simulink model "Sanepa_overall_model0x2810x29"  (R2024b)
settings: Solver=VariableStepAuto  StartTime=0.0  StopTime=0.7  RelTol=1e-3
undefined symbols (not defined in the file or in its folder): D11, Delta, DiscIntNeverNeededParam
libraries: spsSeriesRLCLoadLib x69, spsThreePhaseTransformerTwoWindingsLib x23, spsThreePhasePISectionLineLib x18, spsRMSLib x6, spsThreePhaseSeriesRLCBranchLib x4, spsThreePhaseVIMeasurementLib x3, spsCurrentMeasurementLib x3, spsVoltageMeasurementLib x3, spsGroundLib x2, spsThreePhaseBreakerLib x2, spsabctodq0Lib x1, spsdq0toabcLib x1
(part 2 of 2)

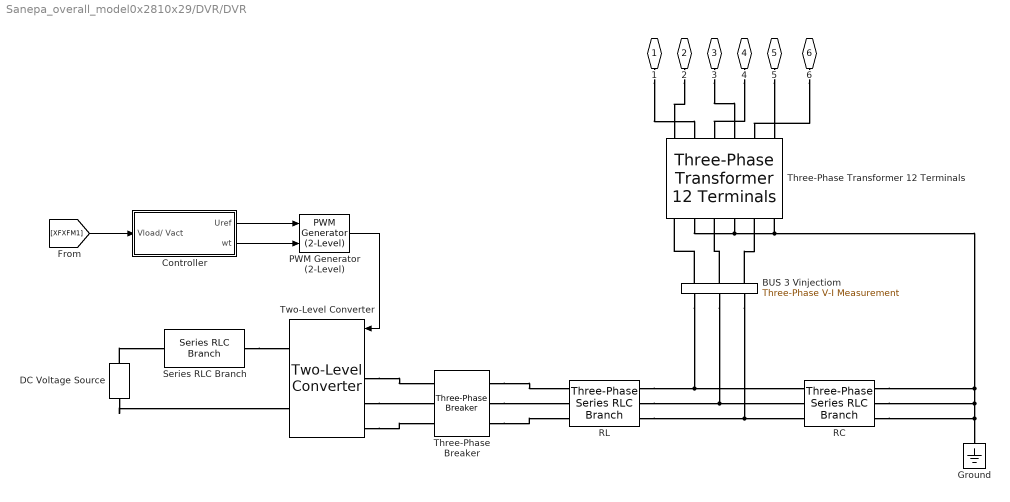
== system Sanepa_overall_model0x2810x29/DVR/DVR ==
  BUS 3 Vinjectiom : spsThreePhaseVIMeasurementLib/Three-Phase V-I Measurement  VoltageMeasurement=phase-to-ground  SetLabelV=on  LabelV=Vinj  Vpu=on  VpuLL=off  CurrentMeasurement=yes  SetLabelI=on  LabelI=Iinj  Ipu=on  Pbase=1e6  Vbase=11000  OutputType=Complex  PhasorSimulation=off  PSBequivalent=0
  Controller : Subsystem
  DC Voltage Source : spsDCVoltageSourceLib/DC Voltage Source  Amplitude=3000  Measurements=None
  Ground : spsGroundLib/Ground  LConnTagsString=a
  PWM Generator (2-Level) : spsPWMGenerator2LevelLib/PWM Generator (2-Level)  ModulatorType=Three-phase bridge (6 pulses)  ModulatorMode=Synchronized  Fc=27*60  Pc=90  nF=2250  MinMax="[ -1  1 ]"  SamplingTechnique=Natural  ModulatingSignals=off  m=0.8  Freq=60  Phase=0  Ts=50e-6  ShowCarrierOutport=off
  RC : spsThreePhaseSeriesRLCBranchLib/Three-Phase Series RLC Branch  LConnTagsString=A|B|C  RConnTagsString=A|B|C  BranchType=RC  Resistance=1  Inductance=1e-3  Capacitance=50e-7  Measurements=None
  RL : spsThreePhaseSeriesRLCBranchLib/Three-Phase Series RLC Branch  LConnTagsString=A|B|C  RConnTagsString=A|B|C  BranchType=L  Resistance=1  Inductance=1e-1  Capacitance=1e-6  Measurements=None
  Series RLC Branch : spsSeriesRLCBranchLib/Series RLC Branch  LConnTagsString=__new0  RConnTagsString=__new0  BranchType=R  Resistance=0.1  Inductance=1e-3  SetiL0=off  InitialCurrent=0  Capacitance=1e-6  Setx0=off  InitialVoltage=0  Measurements=None
  Three-Phase Breaker : spsThreePhaseBreakerLib/Three-Phase Breaker  InitialState=open  SwitchA=on  SwitchB=on  SwitchC=on  SwitchTimes=0  External=off  BreakerResistance=0.01  SnubberResistance=1e6  SnubberCapacitance=inf  Measurements=None
  Three-Phase Transformer 12 Terminals : spsThreePhaseTransformer12TerminalsLib/Three-Phase Transformer 12 Terminals  RatedPower=[ 100e3 50 ]  Winding1="[ 100 0.00001  0.0003 ]"  Winding2=[ 1000 0.00001 0.0003 ]  RmXm=[ 200 200 ]
  Two-Level Converter : spsTwoLevelConverterLib/Two-Level Converter  ModelType=Switching devices  Ron=1e-3  Rs=1e6  Cs=inf  Vforward=[0,0]  Ron_Diode=1e-3  Rs_Diode=1e6  Cs_Diode=inf  Vf_Diode=1e-3  Rs_CurrentSource=inf  Ron_ACsource=1e-3
  1 : PMIOPort  Tag=PMCPort  Side=Left
  2 : PMIOPort  Tag=PMCPort  Port=2  Side=Left
  3 : PMIOPort  Tag=PMCPort  Port=3  Side=Left
  4 : PMIOPort  Tag=PMCPort  Port=4  Side=Left
  5 : PMIOPort  Tag=PMCPort  Port=5  Side=Left
  6 : PMIOPort  Tag=PMCPort  Port=6  Side=Left
  wires:
  PWM Generator (2-Level)/1 -> Two-Level Converter/1
  Controller/1(Uref) -> PWM Generator (2-Level)/1
  Controller/2(wt) -> PWM Generator (2-Level)/2
  [XFXFM1] -> Controller/1(Vload/ Vact)
  connections:
  DC Voltage Source/RConn1 -- Series RLC Branch/LConn1
  DC Voltage Source/LConn1 -- Two-Level Converter/RConn2
  Series RLC Branch/RConn1 -- Two-Level Converter/RConn1
  Two-Level Converter/LConn1 -- Three-Phase Breaker/LConn1
  Two-Level Converter/LConn2 -- Three-Phase Breaker/LConn2
  Two-Level Converter/LConn3 -- Three-Phase Breaker/LConn3
  Three-Phase Breaker/RConn1 -- RL/LConn1
  Three-Phase Breaker/RConn2 -- RL/LConn2
  Three-Phase Breaker/RConn3 -- RL/LConn3
  RL/RConn1 -- BUS 3 Vinjectiom/LConn1 -- RC/LConn1
  RL/RConn2 -- BUS 3 Vinjectiom/LConn2 -- RC/LConn2
  RL/RConn3 -- BUS 3 Vinjectiom/LConn3 -- RC/LConn3
  Three-Phase Transformer 12 Terminals/LConn2 -- Three-Phase Transformer 12 Terminals/LConn4 -- RC/RConn3 -- Ground/LConn1 -- RC/RConn2 -- RC/RConn1 -- Three-Phase Transformer 12 Terminals/LConn6
  BUS 3 Vinjectiom/RConn1 -- Three-Phase Transformer 12 Terminals/LConn1
  BUS 3 Vinjectiom/RConn2 -- Three-Phase Transformer 12 Terminals/LConn3
  BUS 3 Vinjectiom/RConn3 -- Three-Phase Transformer 12 Terminals/LConn5
  1/RConn1 -- Three-Phase Transformer 12 Terminals/RConn2
  2/RConn1 -- Three-Phase Transformer 12 Terminals/RConn1
  3/RConn1 -- Three-Phase Transformer 12 Terminals/RConn4
  4/RConn1 -- Three-Phase Transformer 12 Terminals/RConn3
  5/RConn1 -- Three-Phase Transformer 12 Terminals/RConn6
  6/RConn1 -- Three-Phase Transformer 12 Terminals/RConn5

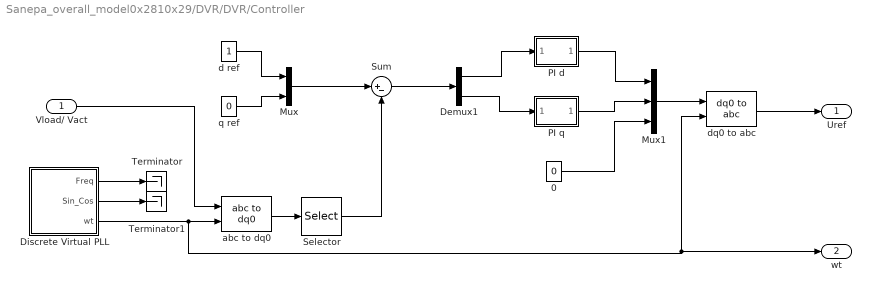
== system Sanepa_overall_model0x2810x29/DVR/DVR/Controller ==
  Vload/ Vact : Inport
  0 : Constant  Value=0
  Demux1 : Demux  Outputs=2
  Discrete Virtual PLL : Subsystem  DialogController=POWERSYS.PowerSysDialog  mask(Discrete Virtual PLL){Freq=50, Phase=30, Ts=50e-6}
      mask prompts: Freq "Frequency (Hz):"; Phase "Phase (degrees):"; Ts "Sample time:"
      mask help:
      | This virtual PLL has no input signal. The block simulates the outputs of an actual PLL by  using the parameters specified in the mask.
      |
      | Output 1: Frequency (Hz)
      | Output 2: Vectorized output  [sin(wt)  cos(wt)]
      | Output 3: wt in rad/s (varying from 0 to 2*pi)
      mask init:
      | power_initmask();
      mask Display: disp('')
  Mux : Mux  Inputs=2
  Mux1 : Mux  Inputs=3
  "PI d " : Subsystem  DialogController=POWERSYS.PowerSysDialog  mask(Discrete PI Controller){Kp=35, Ki=120, Par_Limits=[inf -inf], Init=0, Ts=50e-6}
      mask prompts: Kp "Proportional gain (Kp):"; Ki "Integral gain (Ki):"; Par_Limits "Output limits: [ Upper   Lower ]"; Init "Output initial value:"; Ts "Sample time:"
      mask help: This block implements a discrete PI controller.
      mask init:
      | UpperLimit=Par_Limits(1);
      | LowerLimit=Par_Limits(2);
      | power_initmask();
      mask Display: disp('PI');
  PI q : Subsystem  DialogController=POWERSYS.PowerSysDialog  mask(Discrete PI Controller){Kp=20, Ki=220, Par_Limits=[inf -inf], Init=0, Ts=50e-6}
      mask prompts: Kp "Proportional gain (Kp):"; Ki "Integral gain (Ki):"; Par_Limits "Output limits: [ Upper   Lower ]"; Init "Output initial value:"; Ts "Sample time:"
      mask help: This block implements a discrete PI controller.
      mask init:
      | UpperLimit=Par_Limits(1);
      | LowerLimit=Par_Limits(2);
      | power_initmask();
      mask Display: disp('PI');
  Selector : Selector  InputPortWidth=3  IndexOptions=Index vector (dialog)  Indices=[1 2]  OutputSizes=1
  Sum : Sum  Inputs=|+-
  Terminator : Terminator
  Terminator1 : Terminator
  abc to dq0 : spsabctodq0Lib/abc to dq0  Alignment=90 degrees behind phase A axis
  d ref : Constant
  dq0 to abc : spsdq0toabcLib/dq0 to abc  Alignment=90 degrees behind phase A axis
  q ref : Constant  Value=0
  Uref : Outport  VectorParamsAs1DForOutWhenUnconnected=off
  wt : Outport  Port=2  VectorParamsAs1DForOutWhenUnconnected=off
  wires:
  Discrete Virtual PLL/1(Freq) -> Terminator/1
  Discrete Virtual PLL/2(Sin_Cos) -> Terminator1/1
  Discrete Virtual PLL/3(wt) -> wt/1, dq0 to abc/2, abc to dq0/2
  Vload/ Vact/1 -> abc to dq0/1
  abc to dq0/1 -> Selector/1
  Selector/1 -> Sum/2
  Mux/1 -> Sum/1
  q ref/1 -> Mux/2
  d ref/1 -> Mux/1
  Sum/1 -> Demux1/1
  Demux1/1 -> "PI d "/1(Error)
  Demux1/2 -> PI q/1(Error)
  "PI d "/1(Out) -> Mux1/1
  PI q/1(Out) -> Mux1/2
  Mux1/1 -> dq0 to abc/1
  dq0 to abc/1 -> Uref/1
  0/1 -> Mux1/3

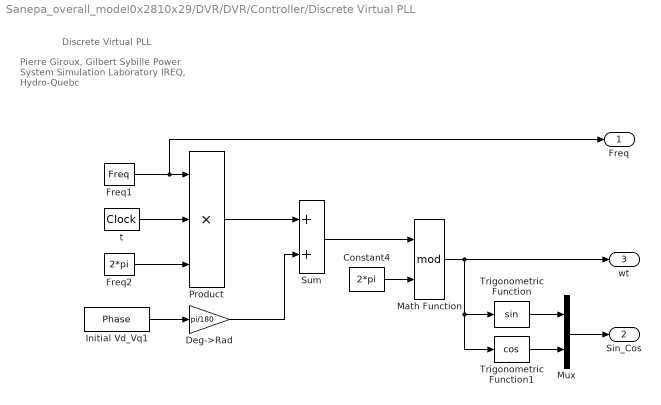
== system Sanepa_overall_model0x2810x29/DVR/DVR/Controller/Discrete Virtual PLL ==
  note: Pierre Giroux, Gilbert Sybille
      | Power System Simulation Laboratory
      | IREQ, Hydro-Quebc
  note: Discrete Virtual PLL
  Constant4 : Constant  Value=2*pi
  Deg->Rad : Gain  Gain=pi/180  SaturateOnIntegerOverflow=on  OutDataTypeStr=Inherit: Same as input  ParamDataTypeStr=Inherit: Same as input
  Freq1 : Constant  Value=Freq
  Freq2 : Constant  Value=2*pi
  Initial Vd_Vq1 : Constant  Value=Phase
  Math Function : Math  Operator=mod  SignedPower=on
  Mux : Mux  Inputs=2
  Product : Product  Inputs=***  InputSameDT=on  SaturateOnIntegerOverflow=on  OutDataTypeStr=Inherit: Same as first input
  Sum : Sum  InputSameDT=on  SaturateOnIntegerOverflow=on  OutDataTypeStr=Inherit: Same as first input
  Trigonometric Function : Trigonometry
  Trigonometric Function1 : Trigonometry  Operator=cos
  t : DigitalClock  SampleTime=Ts
  Freq : Outport  VectorParamsAs1DForOutWhenUnconnected=off
  Sin_Cos : Outport  Port=2  VectorParamsAs1DForOutWhenUnconnected=off
  wt : Outport  Port=3  VectorParamsAs1DForOutWhenUnconnected=off
  wires:
  Sum/1 -> Math Function/1
  t/1 -> Product/2
  Freq2/1 -> Product/3
  Freq1/1 -> Product/1, Freq/1
  Deg->Rad/1 -> Sum/2
  Initial Vd_Vq1/1 -> Deg->Rad/1
  Product/1 -> Sum/1
  Constant4/1 -> Math Function/2
  Math Function/1 -> wt/1, Trigonometric Function1/1, Trigonometric Function/1
  Trigonometric Function/1 -> Mux/1
  Trigonometric Function1/1 -> Mux/2
  Mux/1 -> Sin_Cos/1

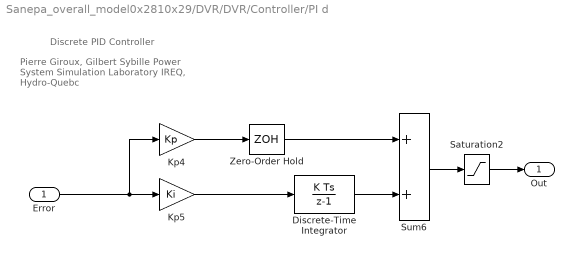
== system Sanepa_overall_model0x2810x29/DVR/DVR/Controller/PI d  ==
  note: Discrete PID Controller
  note: Pierre Giroux, Gilbert Sybille
      | Power System Simulation Laboratory
      | IREQ, Hydro-Quebc
  Error : Inport  SampleTime=Ts
  Discrete-Time Integrator : DiscreteIntegrator  InitialCondition=Init  SampleTime=Ts  LimitOutput=on  UpperSaturationLimit=UpperLimit  LowerSaturationLimit=LowerLimit  ICPrevOutput=DiscIntNeverNeededParam  ICPrevScaledInput=DiscIntNeverNeededParam
  Kp4 : Gain  Gain=Kp  SaturateOnIntegerOverflow=on  SampleTime=Ts  OutDataTypeStr=Inherit: Same as input  ParamDataTypeStr=Inherit: Same as input
  Kp5 : Gain  Gain=Ki  SaturateOnIntegerOverflow=on  SampleTime=Ts  OutDataTypeStr=Inherit: Same as input  ParamDataTypeStr=Inherit: Same as input
  Saturation2 : Saturate  UpperLimit=UpperLimit  LowerLimit=LowerLimit  SampleTime=Ts
  Sum6 : Sum  InputSameDT=on  SaturateOnIntegerOverflow=on  SampleTime=Ts  OutDataTypeStr=Inherit: Same as first input
  Zero-Order Hold : ZeroOrderHold  SampleTime=Ts
  Out : Outport  SampleTime=Ts  InitialOutput=0  VectorParamsAs1DForOutWhenUnconnected=off
  wires:
  Zero-Order Hold/1 -> Sum6/1
  Saturation2/1 -> Out/1
  Discrete-Time Integrator/1 -> Sum6/2
  Kp4/1 -> Zero-Order Hold/1
  Kp5/1 -> Discrete-Time Integrator/1
  Sum6/1 -> Saturation2/1
  Error/1 -> Kp5/1, Kp4/1

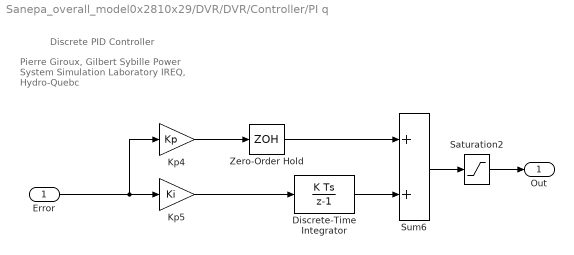
== system Sanepa_overall_model0x2810x29/DVR/DVR/Controller/PI q ==
  note: Pierre Giroux, Gilbert Sybille
      | Power System Simulation Laboratory
      | IREQ, Hydro-Quebc
  note: Discrete PID Controller
  Error : Inport  SampleTime=Ts
  Discrete-Time Integrator : DiscreteIntegrator  InitialCondition=Init  SampleTime=Ts  LimitOutput=on  UpperSaturationLimit=UpperLimit  LowerSaturationLimit=LowerLimit  ICPrevOutput=DiscIntNeverNeededParam  ICPrevScaledInput=DiscIntNeverNeededParam
  Kp4 : Gain  Gain=Kp  SaturateOnIntegerOverflow=on  SampleTime=Ts  OutDataTypeStr=Inherit: Same as input  ParamDataTypeStr=Inherit: Same as input
  Kp5 : Gain  Gain=Ki  SaturateOnIntegerOverflow=on  SampleTime=Ts  OutDataTypeStr=Inherit: Same as input  ParamDataTypeStr=Inherit: Same as input
  Saturation2 : Saturate  UpperLimit=UpperLimit  LowerLimit=LowerLimit  SampleTime=Ts
  Sum6 : Sum  InputSameDT=on  SaturateOnIntegerOverflow=on  SampleTime=Ts  OutDataTypeStr=Inherit: Same as first input
  Zero-Order Hold : ZeroOrderHold  SampleTime=Ts
  Out : Outport  SampleTime=Ts  InitialOutput=0  VectorParamsAs1DForOutWhenUnconnected=off
  wires:
  Error/1 -> Kp4/1, Kp5/1
  Sum6/1 -> Saturation2/1
  Kp5/1 -> Discrete-Time Integrator/1
  Kp4/1 -> Zero-Order Hold/1
  Discrete-Time Integrator/1 -> Sum6/2
  Saturation2/1 -> Out/1
  Zero-Order Hold/1 -> Sum6/1
